simulink model "eightenPulseRectifier"  (R2024a)
settings: Solver=VariableStepAuto  StartTime=0.0  StopTime=.1  MaxStep=.00001  RelTol=1e-3
undefined symbols (not defined in the file): D1, lagging, pulse
libraries: spsVoltageMeasurementLib x34, spsControlledVoltageSourceLib x9, spsUniversalBridgeLib x9, spsSeriesRLCBranchLib x6, spsZigzagPhaseShiftingTransformerLib x6, spsGroundLib x5, spsThreePhaseTransformerTwoWindingsLib x3, spsPulseGeneratorThyristor6PulseLib x2, spsPLLLib x1, spsPLL3phLib x1, spsRMSLib x1, spsThreePhaseVIMeasurementLib x1
settings Model: Creator=User  LastModifiedBy=User

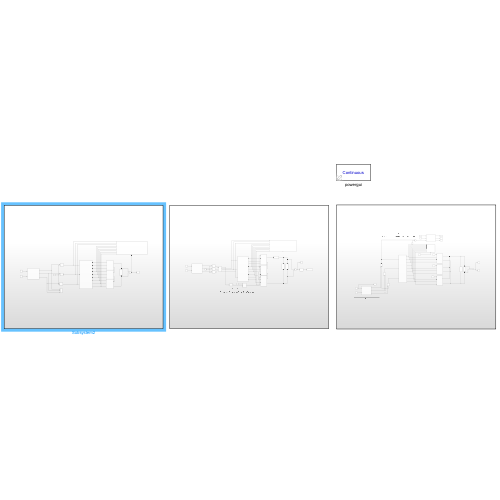
[thumbnail: Simulink's stored preview of the top-level diagram]
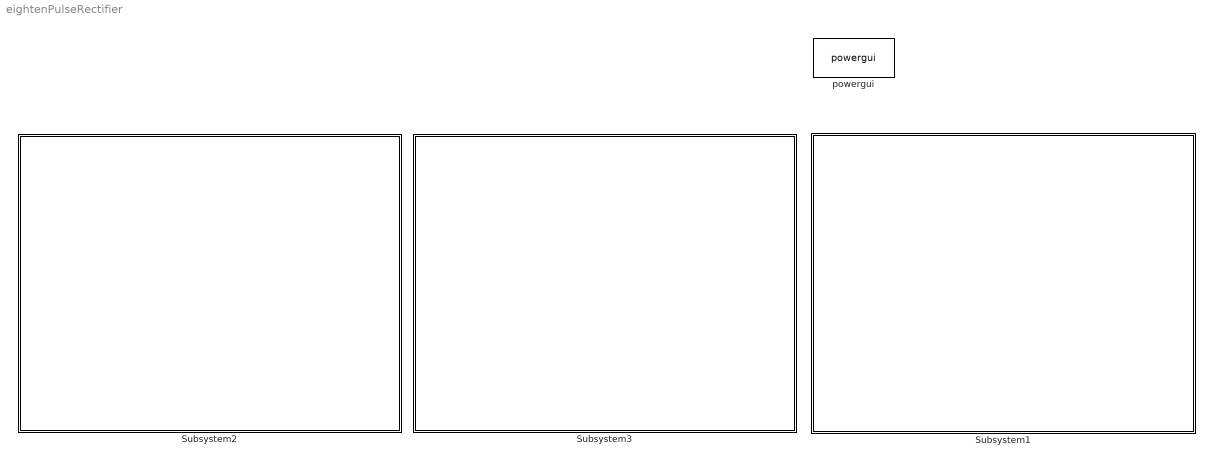
== system eightenPulseRectifier ==
  Subsystem1 : Subsystem
  Subsystem2 : Subsystem
  Subsystem3 : Subsystem
  powergui : sps_lib/powergui  Priority=1  SimulationMode=Continuous  SampleTime=50e-6  frequency=60  Iterations=50  frequencyindice=0  Pbase=100e6  ErrMax=1e-4  UnitsV=kV  UnitsW=MW  buscounter=0  FunctionMessages=off  echomessages=off  EnableUseOfTLC=off  CurrentSourceSwitches=off  DisableSnubberDevices=off  DisableRonSwitches=off  DisableVfSwitches=off  DisplayEquations=off  AutomaticDiscreteSolvers=off  SolverType=Tustin/Backward Euler (TBE)  Interpol=off  ExternalGateDelay=off  methode=off  Ts=100  x0status=blocks  SPID=on  SwTol=0  HookPort=off  NonlinearTolerance=1e-4  nMaxIteration=100  ContinueOnMaxIteration=off  RestoreLinks=warning  ResistiveCurrentMeasurement=off  Frange=[0:2:500]  Ylog=off  Xlog=on  ShowGrid=off  save=off  variable=ZData  structure=0  ZoomFFT=off  StartTime=0.0  cycles=1  DisplayStyle=1  fundamental=60  FreqAxis=off  MaxFrequency=1000  frequencyindicesteady=1  RmsSteady=1  display=off

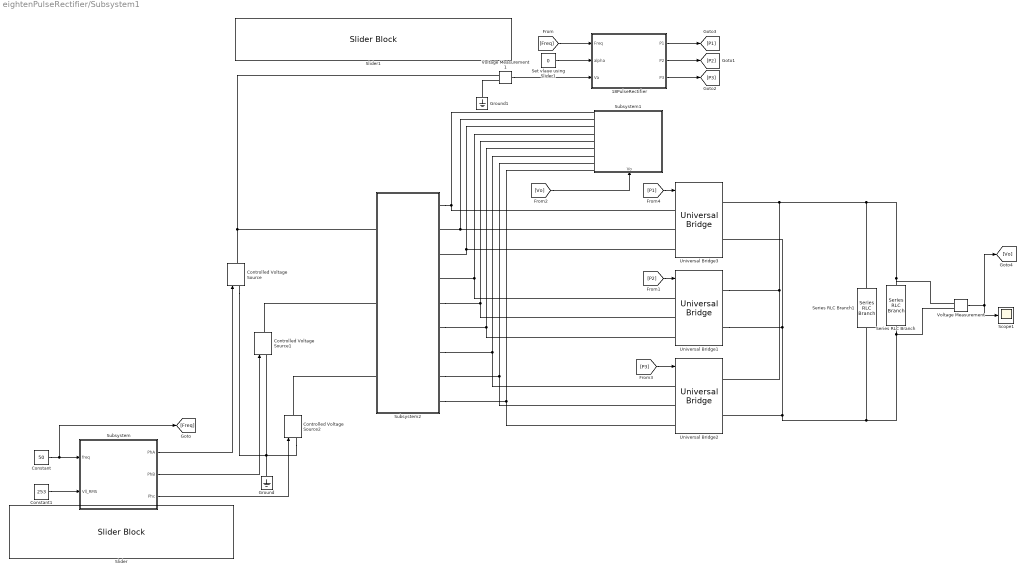
== system eightenPulseRectifier/Subsystem1 ==
  18PulseRectifier : Subsystem
  Constant : Constant  Value=50
  Constant1 : Constant  Value=253
  Controlled Voltage Source : spsControlledVoltageSourceLib/Controlled Voltage Source  Initialize=on  Source_Type=AC  Amplitude=0  Phase=0  Frequency=0  Measurements=None
  Controlled Voltage Source1 : spsControlledVoltageSourceLib/Controlled Voltage Source  Initialize=on  Source_Type=AC  Amplitude=0  Phase=0  Frequency=0  Measurements=None
  Controlled Voltage Source2 : spsControlledVoltageSourceLib/Controlled Voltage Source  Initialize=on  Source_Type=AC  Amplitude=0  Phase=0  Frequency=0  Measurements=None
  Ground : spsGroundLib/Ground  LConnTagsString=a
  Ground1 : spsGroundLib/Ground  LConnTagsString=a
  Scope1 : Scope
  Series RLC Branch : spsSeriesRLCBranchLib/Series RLC Branch  LConnTagsString=__new0  RConnTagsString=__new0  BranchType=R  Resistance=1  Inductance=1e-3  SetiL0=off  InitialCurrent=0  Capacitance=1e-6  Setx0=off  InitialVoltage=0  Measurements=None
  Series RLC Branch1 : spsSeriesRLCBranchLib/Series RLC Branch  LConnTagsString=__new0  RConnTagsString=__new0  BranchType=C  Resistance=1  Inductance=1e-3  SetiL0=off  InitialCurrent=0  Capacitance=1e-6  Setx0=off  InitialVoltage=0  Measurements=None
  Set vlaue using Slider1 : Constant  Value=0
  Slider : SliderBlock  ScaleMin=187  ScaleMax=253
  Slider1 : SliderBlock  ScaleMax=150  TickInterval=5
  Subsystem : Subsystem
  Subsystem1 : Subsystem
      settings: PortSchema="{\"entries\":[{\"content\":{\"sides\":[{\"content\":{\"connectorIds\":[\"LConn1\",\"LConn2\",\"LConn3\",\"LConn4\",\"LConn5\",\"LConn6\",\"LConn7\",\"LConn8\",\"LConn9\"]},\"type\":\"ConnectorPlacement.EquallySpacedRectSide\",\"uuid\":\"c528b960-0f89-4916-bc59-feafc106a6fa\"},{\"content\":{\"side\":\"RIGHT\"},\"type\":\"ConnectorPlacement.EquallySpacedRectSide\",\"uuid\":\"71a864a5-f7f4-48a7-95f9-d8a7d95b84d2\"},{\"content\":{\"side\":\"TOP\"},\"type\":\"ConnectorPlacement.EquallySpacedRectSide\",\"uuid\":\"57c5c08c-8233-4b40-a9fb-e09e67286da5\"},{\"content\":{\"connectorIds\":[\"In1\"],\"side\":\"BOTTOM\"},\"type\":\"ConnectorPlacement.EquallySpacedRectSide\",\"uuid\":\"030adcd8-0531-402c-81c9-62e294f4d5af\"}]},\"type\":\"ConnectorPlacement.EquallySpacedConnector\",\"uuid\":\"216ad3eb-0ca6-4d39-b862-04814928268f\"}],\"packageUris\":[\"http://schema.mathworks.com/mf0/Connector/R2020b\"],\"version\":\"1.0\"}"
  Subsystem2 : Subsystem
  Universal Bridge1 : spsUniversalBridgeLib/Universal Bridge  Arms=3  SnubberResistance=1e5  SnubberCapacitance=inf  Device=Thyristors  Ron=1e-3  Lon=0  ForwardVoltages="[  0  0  ]"  ForwardVoltage=0  GTOparameters=[ 10e-6 , 20e-6 ]  IGBTparameters=[ 1e-6 , 2e-6 ]  Measurements=None  Measurements_2=None  converterType=Rectifier
  Universal Bridge2 : spsUniversalBridgeLib/Universal Bridge  Arms=3  SnubberResistance=1e5  SnubberCapacitance=inf  Device=Thyristors  Ron=1e-3  Lon=0  ForwardVoltages="[  0  0  ]"  ForwardVoltage=0  GTOparameters=[ 10e-6 , 20e-6 ]  IGBTparameters=[ 1e-6 , 2e-6 ]  Measurements=None  Measurements_2=None  converterType=Rectifier
  Universal Bridge3 : spsUniversalBridgeLib/Universal Bridge  Arms=3  SnubberResistance=1e5  SnubberCapacitance=inf  Device=Thyristors  Ron=1e-3  Lon=0  ForwardVoltages="[  0  0  ]"  ForwardVoltage=0  GTOparameters=[ 10e-6 , 20e-6 ]  IGBTparameters=[ 1e-6 , 2e-6 ]  Measurements=None  Measurements_2=None  converterType=Rectifier
  Voltage Measurement : spsVoltageMeasurementLib/Voltage Measurement  PhasorSimulation=off  OutputType=Complex  PSBequivalent=0
  Voltage Measurement1 : spsVoltageMeasurementLib/Voltage Measurement  PhasorSimulation=off  OutputType=Complex  PSBequivalent=0
  wires:
  Constant/1 -> [Freq], Subsystem/1(freq)
  Constant1/1 -> Subsystem/2(Vll_RMS)
  Subsystem/3(Phc) -> Controlled Voltage Source2/1
  Subsystem/2(PhB) -> Controlled Voltage Source1/1
  Subsystem/1(PhA) -> Controlled Voltage Source/1
  [P3] -> Universal Bridge2/1
  [Freq] -> 18PulseRectifier/1(Freq)
  18PulseRectifier/1(P1) -> [P1]
  18PulseRectifier/2(P2) -> [P2]
  18PulseRectifier/3(P3) -> [P3]
  Set vlaue using Slider1/1 -> 18PulseRectifier/2(alpha)
  Voltage Measurement/1 -> Scope1/1, [Vo]
  [Vo] -> Subsystem1/1(Vo)
  [P1] -> Universal Bridge3/1
  [P2] -> Universal Bridge1/1
  Voltage Measurement1/1 -> 18PulseRectifier/3(Va)
  connections:
  Subsystem1/LConn9 -- Universal Bridge2/LConn3 -- Subsystem2/RConn9
  Subsystem1/LConn6 -- Universal Bridge1/LConn3 -- Subsystem2/RConn6
  Controlled Voltage Source/RConn1 -- Voltage Measurement1/LConn1 -- Subsystem2/LConn1
  Subsystem1/LConn5 -- Universal Bridge1/LConn2 -- Subsystem2/RConn5
  Subsystem1/LConn7 -- Universal Bridge2/LConn1 -- Subsystem2/RConn7
  Subsystem1/LConn3 -- Subsystem2/RConn3 -- Universal Bridge3/LConn3
  Ground/LConn1 -- Controlled Voltage Source1/LConn1 -- Controlled Voltage Source/LConn1 -- Controlled Voltage Source2/LConn1
  Subsystem1/LConn2 -- Subsystem2/RConn2 -- Universal Bridge3/LConn2
  Voltage Measurement/LConn1 -- Series RLC Branch1/LConn1 -- Universal Bridge2/RConn1 -- Universal Bridge1/RConn1 -- Universal Bridge3/RConn1 -- Series RLC Branch/LConn1
  Series RLC Branch/RConn1 -- Universal Bridge1/RConn2 -- Universal Bridge3/RConn2 -- Universal Bridge2/RConn2 -- Series RLC Branch1/RConn1 -- Voltage Measurement/LConn2
  Subsystem1/LConn8 -- Universal Bridge2/LConn2 -- Subsystem2/RConn8
  Subsystem1/LConn4 -- Universal Bridge1/LConn1 -- Subsystem2/RConn4
  Controlled Voltage Source2/RConn1 -- Subsystem2/LConn3
  Controlled Voltage Source1/RConn1 -- Subsystem2/LConn2
  Subsystem1/LConn1 -- Universal Bridge3/LConn1 -- Subsystem2/RConn1
  Ground1/LConn1 -- Voltage Measurement1/LConn2

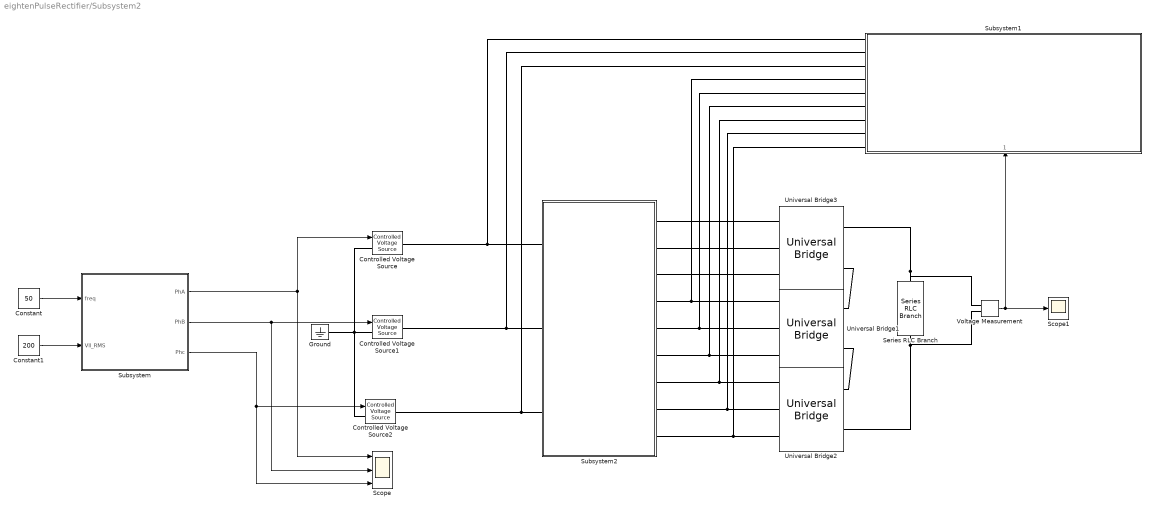
== system eightenPulseRectifier/Subsystem2 ==
  Constant : Constant  Value=50
  Constant1 : Constant  Value=200
  Controlled Voltage Source : spsControlledVoltageSourceLib/Controlled Voltage Source  Initialize=on  Source_Type=AC  Amplitude=0  Phase=0  Frequency=0  Measurements=None
  Controlled Voltage Source1 : spsControlledVoltageSourceLib/Controlled Voltage Source  Initialize=on  Source_Type=AC  Amplitude=0  Phase=0  Frequency=0  Measurements=None
  Controlled Voltage Source2 : spsControlledVoltageSourceLib/Controlled Voltage Source  Initialize=on  Source_Type=AC  Amplitude=0  Phase=0  Frequency=0  Measurements=None
  Ground : spsGroundLib/Ground  LConnTagsString=a
  Scope : Scope  NumInputPorts=3
  Scope1 : Scope
  Series RLC Branch : spsSeriesRLCBranchLib/Series RLC Branch  LConnTagsString=__new0  RConnTagsString=__new0  BranchType=R  Resistance=20  Inductance=1e-3  SetiL0=off  InitialCurrent=0  Capacitance=1e-6  Setx0=off  InitialVoltage=0  Measurements=None
  Subsystem : Subsystem
  Subsystem1 : Subsystem
      settings: PortSchema="{\"entries\":[{\"content\":{\"sides\":[{\"content\":{\"connectorIds\":[\"LConn1\",\"LConn2\",\"LConn3\",\"LConn4\",\"LConn5\",\"LConn6\",\"LConn7\",\"LConn8\",\"LConn9\"]},\"type\":\"ConnectorPlacement.EquallySpacedRectSide\",\"uuid\":\"c528b960-0f89-4916-bc59-feafc106a6fa\"},{\"content\":{\"side\":\"RIGHT\"},\"type\":\"ConnectorPlacement.EquallySpacedRectSide\",\"uuid\":\"71a864a5-f7f4-48a7-95f9-d8a7d95b84d2\"},{\"content\":{\"side\":\"TOP\"},\"type\":\"ConnectorPlacement.EquallySpacedRectSide\",\"uuid\":\"57c5c08c-8233-4b40-a9fb-e09e67286da5\"},{\"content\":{\"connectorIds\":[\"In1\"],\"side\":\"BOTTOM\"},\"type\":\"ConnectorPlacement.EquallySpacedRectSide\",\"uuid\":\"f6f9f7ac-8837-43ce-91db-f6801ff1a468\"}]},\"type\":\"ConnectorPlacement.EquallySpacedConnector\",\"uuid\":\"216ad3eb-0ca6-4d39-b862-04814928268f\"}],\"packageUris\":[\"http://schema.mathworks.com/mf0/Connector/R2020b\"],\"version\":\"1.0\"}"
  Subsystem2 : Subsystem
  Universal Bridge1 : spsUniversalBridgeLib/Universal Bridge  Arms=3  SnubberResistance=1e5  SnubberCapacitance=inf  Device=Diodes  Ron=1e-3  Lon=0  ForwardVoltages="[  0  0  ]"  ForwardVoltage=0  GTOparameters=[ 10e-6 , 20e-6 ]  IGBTparameters=[ 1e-6 , 2e-6 ]  Measurements=None  Measurements_2=None  converterType=Rectifier
  Universal Bridge2 : spsUniversalBridgeLib/Universal Bridge  Arms=3  SnubberResistance=1e5  SnubberCapacitance=inf  Device=Diodes  Ron=1e-3  Lon=0  ForwardVoltages="[  0  0  ]"  ForwardVoltage=0  GTOparameters=[ 10e-6 , 20e-6 ]  IGBTparameters=[ 1e-6 , 2e-6 ]  Measurements=None  Measurements_2=None  converterType=Rectifier
  Universal Bridge3 : spsUniversalBridgeLib/Universal Bridge  Arms=3  SnubberResistance=1e5  SnubberCapacitance=inf  Device=Diodes  Ron=1e-3  Lon=0  ForwardVoltages="[  0  0  ]"  ForwardVoltage=0  GTOparameters=[ 10e-6 , 20e-6 ]  IGBTparameters=[ 1e-6 , 2e-6 ]  Measurements=None  Measurements_2=None  converterType=Rectifier
  Voltage Measurement : spsVoltageMeasurementLib/Voltage Measurement  PhasorSimulation=off  OutputType=Complex  PSBequivalent=0
  wires:
  Subsystem/1(PhA) -> Controlled Voltage Source/1, Scope/1
  Subsystem/2(PhB) -> Scope/2, Controlled Voltage Source1/1
  Subsystem/3(Phc) -> Scope/3, Controlled Voltage Source2/1
  Constant1/1 -> Subsystem/2(Vll_RMS)
  Constant/1 -> Subsystem/1(freq)
  Voltage Measurement/1 -> Scope1/1, Subsystem1/1(" ")
  connections:
  Subsystem2/RConn3 -- Universal Bridge3/LConn3
  Subsystem2/RConn2 -- Universal Bridge3/LConn2
  Subsystem2/RConn1 -- Universal Bridge3/LConn1
  Subsystem2/RConn7 -- Subsystem1/LConn7 -- Universal Bridge2/LConn1
  Subsystem1/LConn2 -- Subsystem2/LConn2 -- Controlled Voltage Source1/RConn1
  Subsystem2/RConn9 -- Subsystem1/LConn9 -- Universal Bridge2/LConn3
  Subsystem2/RConn6 -- Universal Bridge1/LConn3 -- Subsystem1/LConn6
  Subsystem2/LConn1 -- Controlled Voltage Source/RConn1 -- Subsystem1/LConn1
  Subsystem2/LConn3 -- Controlled Voltage Source2/RConn1 -- Subsystem1/LConn3
  Subsystem2/RConn8 -- Subsystem1/LConn8 -- Universal Bridge2/LConn2
  Subsystem2/RConn4 -- Universal Bridge1/LConn1 -- Subsystem1/LConn4
  Controlled Voltage Source1/LConn1 -- Controlled Voltage Source2/LConn1 -- Ground/LConn1 -- Controlled Voltage Source/LConn1
  Subsystem2/RConn5 -- Universal Bridge1/LConn2 -- Subsystem1/LConn5
  Voltage Measurement/LConn1 -- Universal Bridge3/RConn1 -- Series RLC Branch/LConn1
  Universal Bridge3/RConn2 -- Universal Bridge1/RConn1
  Universal Bridge1/RConn2 -- Universal Bridge2/RConn1
  Voltage Measurement/LConn2 -- Universal Bridge2/RConn2 -- Series RLC Branch/RConn1

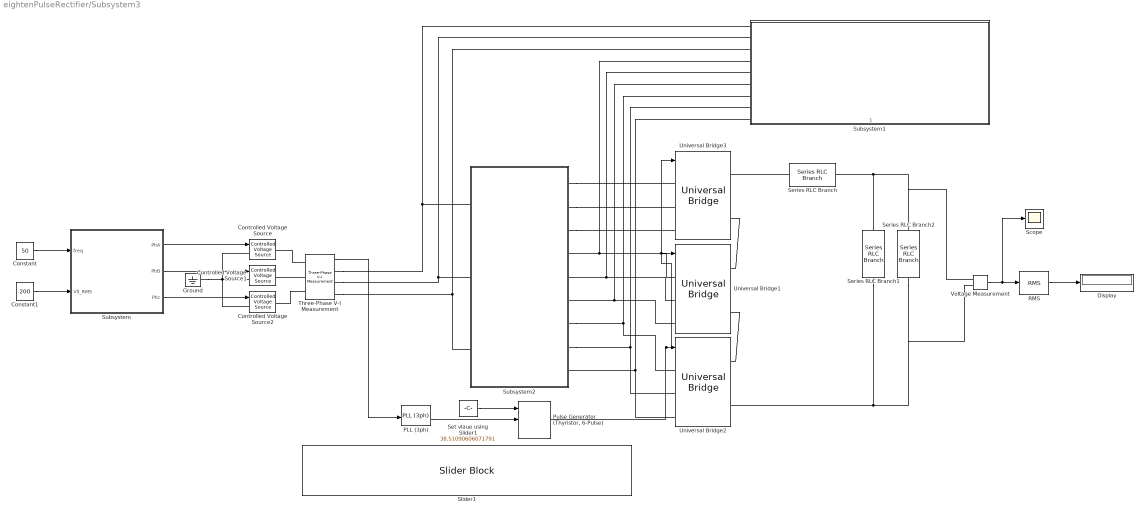
== system eightenPulseRectifier/Subsystem3 ==
  Constant : Constant  Value=50
  Constant1 : Constant  Value=200
  Controlled Voltage Source : spsControlledVoltageSourceLib/Controlled Voltage Source  Initialize=on  Source_Type=AC  Amplitude=0  Phase=0  Frequency=0  Measurements=None
  Controlled Voltage Source1 : spsControlledVoltageSourceLib/Controlled Voltage Source  Initialize=on  Source_Type=AC  Amplitude=0  Phase=0  Frequency=0  Measurements=None
  Controlled Voltage Source2 : spsControlledVoltageSourceLib/Controlled Voltage Source  Initialize=on  Source_Type=AC  Amplitude=0  Phase=0  Frequency=0  Measurements=None
  Display : Display
  Ground : spsGroundLib/Ground  LConnTagsString=a
  PLL (3ph) : spsPLL3phLib/PLL (3ph)  Fmin=45  Par_Init=[0, 60]  ParK=[180, 3200, 1]  TcD=1e-4  MaxRateChangeFreq=12  FilterCutOffFreq=25  Ts=0  AGC=on
  "Pulse Generator (Thyristor, 6-Pulse)" : spsPulseGeneratorThyristor6PulseLib/Pulse Generator (Thyristor, 6-Pulse)  GenType=6-pulse  Delta=D1 (lagging)  pwidth=120  Double_Pulse=off  Ts=0
      settings: LibrarySourceBlock=|
      | sps_lib/Power Electronics/Power Electronics Control/Pulse Generator
      | (Thyristor, 6-Pulse)
  RMS : spsRMSLib/RMS  TrueRMS=on  Freq=50  RMSInit=120  Ts=0
  Scope : Scope
  Series RLC Branch : spsSeriesRLCBranchLib/Series RLC Branch  LConnTagsString=__new0  RConnTagsString=__new0  BranchType=L  Resistance=1  Inductance=200e-3  SetiL0=off  InitialCurrent=0  Capacitance=1e-6  Setx0=off  InitialVoltage=0  Measurements=None
  Series RLC Branch1 : spsSeriesRLCBranchLib/Series RLC Branch  LConnTagsString=__new0  RConnTagsString=__new0  BranchType=C  Resistance=1  Inductance=200e-3  SetiL0=off  InitialCurrent=0  Capacitance=10e-6  Setx0=off  InitialVoltage=0  Measurements=None
  Series RLC Branch2 : spsSeriesRLCBranchLib/Series RLC Branch  LConnTagsString=__new0  RConnTagsString=__new0  BranchType=R  Resistance=1400  Inductance=200e-3  SetiL0=off  InitialCurrent=0  Capacitance=10e-6  Setx0=off  InitialVoltage=0  Measurements=None
  Set vlaue using Slider1 : Constant  Value=38.51090606071791
  Slider1 : SliderBlock  ScaleMax=150  TickInterval=5
  Subsystem : Subsystem
  Subsystem1 : Subsystem
      settings: PortSchema="{\"entries\":[{\"content\":{\"sides\":[{\"content\":{\"connectorIds\":[\"LConn1\",\"LConn2\",\"LConn3\",\"LConn4\",\"LConn5\",\"LConn6\",\"LConn7\",\"LConn8\",\"LConn9\"]},\"type\":\"ConnectorPlacement.EquallySpacedRectSide\",\"uuid\":\"c528b960-0f89-4916-bc59-feafc106a6fa\"},{\"content\":{\"side\":\"RIGHT\"},\"type\":\"ConnectorPlacement.EquallySpacedRectSide\",\"uuid\":\"71a864a5-f7f4-48a7-95f9-d8a7d95b84d2\"},{\"content\":{\"side\":\"TOP\"},\"type\":\"ConnectorPlacement.EquallySpacedRectSide\",\"uuid\":\"57c5c08c-8233-4b40-a9fb-e09e67286da5\"},{\"content\":{\"connectorIds\":[\"In1\"],\"side\":\"BOTTOM\"},\"type\":\"ConnectorPlacement.EquallySpacedRectSide\",\"uuid\":\"f6f9f7ac-8837-43ce-91db-f6801ff1a468\"}]},\"type\":\"ConnectorPlacement.EquallySpacedConnector\",\"uuid\":\"216ad3eb-0ca6-4d39-b862-04814928268f\"}],\"packageUris\":[\"http://schema.mathworks.com/mf0/Connector/R2020b\"],\"version\":\"1.0\"}"
  Subsystem2 : Subsystem
  Three-Phase V-I Measurement : spsThreePhaseVIMeasurementLib/Three-Phase V-I Measurement  VoltageMeasurement=phase-to-ground  SetLabelV=off  LabelV=Vabc  Vpu=off  VpuLL=off  CurrentMeasurement=no  SetLabelI=off  LabelI=Iabc  Ipu=off  Pbase=100e6  Vbase=500e3  OutputType=Complex  PhasorSimulation=off  PSBequivalent=0
  Universal Bridge1 : spsUniversalBridgeLib/Universal Bridge  Arms=3  SnubberResistance=1e5  SnubberCapacitance=inf  Device=Thyristors  Ron=1e-3  Lon=0  ForwardVoltages="[  0  0  ]"  ForwardVoltage=0  GTOparameters=[ 10e-6 , 20e-6 ]  IGBTparameters=[ 1e-6 , 2e-6 ]  Measurements=None  Measurements_2=None  converterType=Rectifier
  Universal Bridge2 : spsUniversalBridgeLib/Universal Bridge  Arms=3  SnubberResistance=1e5  SnubberCapacitance=inf  Device=Thyristors  Ron=1e-3  Lon=0  ForwardVoltages="[  0  0  ]"  ForwardVoltage=0  GTOparameters=[ 10e-6 , 20e-6 ]  IGBTparameters=[ 1e-6 , 2e-6 ]  Measurements=None  Measurements_2=None  converterType=Rectifier
  Universal Bridge3 : spsUniversalBridgeLib/Universal Bridge  Arms=3  SnubberResistance=1e5  SnubberCapacitance=inf  Device=Thyristors  Ron=1e-3  Lon=0  ForwardVoltages="[  0  0  ]"  ForwardVoltage=0  GTOparameters=[ 10e-6 , 20e-6 ]  IGBTparameters=[ 1e-6 , 2e-6 ]  Measurements=None  Measurements_2=None  converterType=Rectifier
  Voltage Measurement : spsVoltageMeasurementLib/Voltage Measurement  PhasorSimulation=off  OutputType=Complex  PSBequivalent=0
  wires:
  Constant/1 -> Subsystem/1(freq)
  Constant1/1 -> Subsystem/2(Vll_RMS)
  Subsystem/3(Phc) -> Controlled Voltage Source2/1
  Subsystem/2(PhB) -> Controlled Voltage Source1/1
  Subsystem/1(PhA) -> Controlled Voltage Source/1
  Three-Phase V-I Measurement/1 -> PLL (3ph)/1
  PLL (3ph)/2 -> "Pulse Generator (Thyristor, 6-Pulse)"/2
  Set vlaue using Slider1/1 -> "Pulse Generator (Thyristor, 6-Pulse)"/1
  "Pulse Generator (Thyristor, 6-Pulse)"/1 -> Universal Bridge3/1, Universal Bridge1/1, Universal Bridge2/1
  Voltage Measurement/1 -> Scope/1, RMS/1
  RMS/1 -> Display/1
  connections:
  Subsystem1/LConn5 -- Universal Bridge1/LConn2 -- Subsystem2/RConn5
  Ground/LConn1 -- Controlled Voltage Source/LConn1 -- Controlled Voltage Source1/LConn1 -- Controlled Voltage Source2/LConn1
  Subsystem1/LConn4 -- Universal Bridge1/LConn1 -- Subsystem2/RConn4
  Subsystem1/LConn8 -- Universal Bridge2/LConn2 -- Subsystem2/RConn8
  Subsystem1/LConn3 -- Subsystem2/LConn3 -- Three-Phase V-I Measurement/RConn3
  Subsystem1/LConn1 -- Three-Phase V-I Measurement/RConn1 -- Subsystem2/LConn1
  Subsystem1/LConn6 -- Universal Bridge1/LConn3 -- Subsystem2/RConn6
  Subsystem1/LConn9 -- Universal Bridge2/LConn3 -- Subsystem2/RConn9
  Subsystem2/LConn2 -- Subsystem1/LConn2 -- Three-Phase V-I Measurement/RConn2
  Subsystem1/LConn7 -- Universal Bridge2/LConn1 -- Subsystem2/RConn7
  Subsystem2/RConn1 -- Universal Bridge3/LConn1
  Subsystem2/RConn2 -- Universal Bridge3/LConn2
  Subsystem2/RConn3 -- Universal Bridge3/LConn3
  Three-Phase V-I Measurement/LConn1 -- Controlled Voltage Source/RConn1
  Three-Phase V-I Measurement/LConn2 -- Controlled Voltage Source1/RConn1
  Three-Phase V-I Measurement/LConn3 -- Controlled Voltage Source2/RConn1
  Universal Bridge3/RConn2 -- Universal Bridge1/RConn1
  Universal Bridge1/RConn2 -- Universal Bridge2/RConn1
  Series RLC Branch/LConn1 -- Universal Bridge3/RConn1
  Series RLC Branch1/LConn1 -- Voltage Measurement/LConn1 -- Series RLC Branch2/LConn1 -- Series RLC Branch/RConn1
  Series RLC Branch1/RConn1 -- Series RLC Branch2/RConn1 -- Voltage Measurement/LConn2 -- Universal Bridge2/RConn2

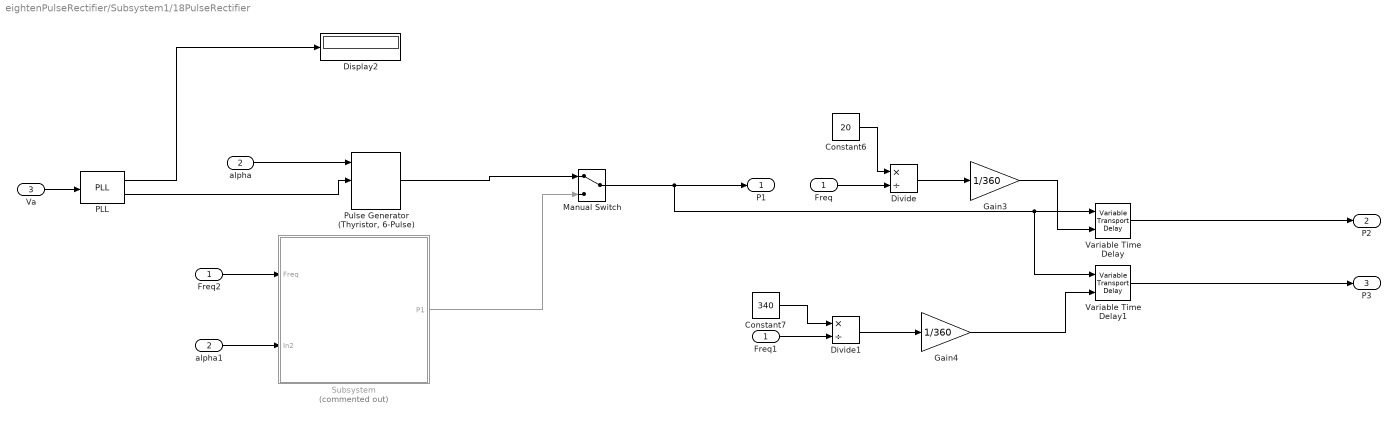
== system eightenPulseRectifier/Subsystem1/18PulseRectifier ==
  Freq : Inport
  alpha : Inport  Port=2
  Va : Inport  Port=3
  Constant6 : Constant  Value=20
  Constant7 : Constant  Value=340
  Display2 : Display
  Divide : Product  Inputs=*/
  Divide1 : Product  Inputs=*/
  Freq1 : InportShadow
  Freq2 : InportShadow
  Gain3 : Gain  Gain=1/360
  Gain4 : Gain  Gain=1/360
  Manual Switch : ManualSwitch
  PLL : spsPLLLib/PLL  Fmin=45  Par_Init=[0, 60]  ParK=[180, 3200, 1]  TcD=1e-4  MaxRateChangeFreq=12  FilterCutOffFreq=25  Ts=0  AGC=on
      settings: LibrarySourceBlock=sps_lib/Control/PLL
  "Pulse Generator (Thyristor, 6-Pulse)" : spsPulseGeneratorThyristor6PulseLib/Pulse Generator (Thyristor, 6-Pulse)  GenType=6-pulse  Delta=D1 (lagging)  pwidth=60  Double_Pulse=off  Ts=0
      settings: LibrarySourceBlock=|
      | sps_lib/Power Electronics/Power Electronics Control/Pulse Generator
      | (Thyristor, 6-Pulse)
  Subsystem : Subsystem  Commented=on
  Variable Time Delay : VariableTransportDelay  MaximumDelay=10
  Variable Time Delay1 : VariableTransportDelay  MaximumDelay=10
  alpha1 : InportShadow  Port=2
  P1 : Outport
  P2 : Outport  Port=2
  P3 : Outport  Port=3
  wires:
  Divide1/1 -> Gain4/1
  Gain4/1 -> Variable Time Delay1/2
  Divide/1 -> Gain3/1
  Gain3/1 -> Variable Time Delay/2
  Variable Time Delay1/1 -> P3/1
  Constant7/1 -> Divide1/1
  Variable Time Delay/1 -> P2/1
  Constant6/1 -> Divide/1
  Freq/1 -> Divide/2
  Freq1/1 -> Divide1/2
  alpha/1 -> "Pulse Generator (Thyristor, 6-Pulse)"/1
  PLL/2 -> "Pulse Generator (Thyristor, 6-Pulse)"/2
  PLL/1 -> Display2/1
  Va/1 -> PLL/1
  Freq2/1 -> Subsystem/1(Freq)
  alpha1/1 -> Subsystem/2(In2)
  Subsystem/1(P1) -> Manual Switch/2
  "Pulse Generator (Thyristor, 6-Pulse)"/1 -> Manual Switch/1
  Manual Switch/1 -> P1/1, Variable Time Delay1/1, Variable Time Delay/1

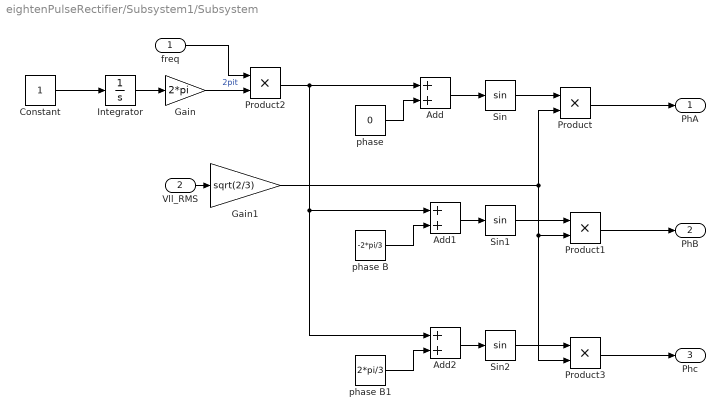
== system eightenPulseRectifier/Subsystem1/Subsystem ==
  freq : Inport
  Vll_RMS : Inport  Port=2
  Add : Sum
  Add1 : Sum
  Add2 : Sum
  Constant : Constant
  Gain : Gain  Gain=2*pi
  Gain1 : Gain  Gain=sqrt(2/3)
  Integrator : Integrator
  Product{,1..3} (4 alike) : Product
  Sin : Trigonometry
  Sin1 : Trigonometry
  Sin2 : Trigonometry
  phase : Constant  Value=0
  phase B : Constant  Value=-2*pi/3
  phase B1 : Constant  Value=2*pi/3
  PhA : Outport
  PhB : Outport  Port=2
  Phc : Outport  Port=3
  wires:
  Sin/1 -> Product/1
  Product3/1 -> Phc/1
  freq/1 -> Product2/1
  Product/1 -> PhA/1
  phase B1/1 -> Add2/2
  Add2/1 -> Sin2/1
  Add1/1 -> Sin1/1
  Add/1 -> Sin/1
  phase B/1 -> Add1/2
  phase/1 -> Add/2
  Vll_RMS/1 -> Gain1/1
  Constant/1 -> Integrator/1
  Integrator/1 -> Gain/1
  Product2/1 -> Add/1, Add1/1, Add2/1
  Product1/1 -> PhB/1
  Sin2/1 -> Product3/1
  Sin1/1 -> Product1/1
  Gain/1 -> Product2/2  "2pit"
  Gain1/1 -> Product1/2, Product3/2, Product/2

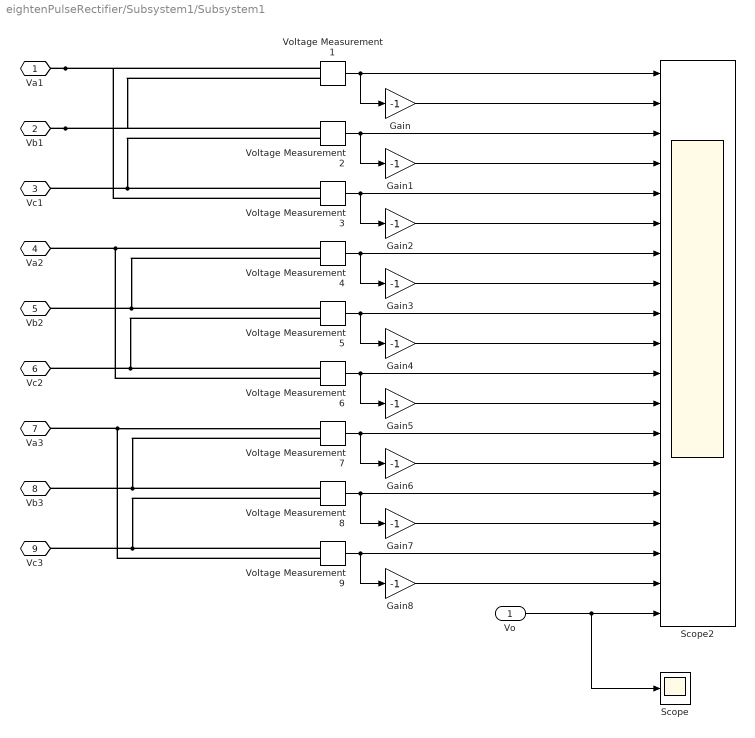
== system eightenPulseRectifier/Subsystem1/Subsystem1 ==
  Vo : Inport
  Gain{,1..8} (9 alike) : Gain  Gain=-1
  Scope : Scope
  Scope2 : Scope  NumInputPorts=19
  Voltage Measurement{1..9} (9 alike) : spsVoltageMeasurementLib/Voltage Measurement  PhasorSimulation=off  OutputType=Complex  PSBequivalent=0
  Va1 : PMIOPort  Side=Left
  Vb1 : PMIOPort  Port=2  Side=Left
  Vc1 : PMIOPort  Port=3  Side=Left
  Va2 : PMIOPort  Port=4  Side=Left
  Vb2 : PMIOPort  Port=5  Side=Left
  Vc2 : PMIOPort  Port=6  Side=Left
  Va3 : PMIOPort  Port=7  Side=Left
  Vb3 : PMIOPort  Port=8  Side=Left
  Vc3 : PMIOPort  Port=9  Side=Left
  wires:
  Voltage Measurement2/1 -> Gain1/1, Scope2/3
  Voltage Measurement4/1 -> Gain3/1, Scope2/7
  Voltage Measurement5/1 -> Gain4/1, Scope2/9
  Voltage Measurement3/1 -> Gain2/1, Scope2/5
  Gain1/1 -> Scope2/4
  Gain8/1 -> Scope2/18
  Gain7/1 -> Scope2/16
  Voltage Measurement9/1 -> Gain8/1, Scope2/17
  Gain5/1 -> Scope2/12
  Voltage Measurement7/1 -> Gain6/1, Scope2/13
  Voltage Measurement6/1 -> Gain5/1, Scope2/11
  Voltage Measurement1/1 -> Gain/1, Scope2/1
  Voltage Measurement8/1 -> Gain7/1, Scope2/15
  Gain4/1 -> Scope2/10
  Gain2/1 -> Scope2/6
  Gain/1 -> Scope2/2
  Gain6/1 -> Scope2/14
  Gain3/1 -> Scope2/8
  Vo/1 -> Scope/1, Scope2/19
  connections:
  Voltage Measurement6/LConn1 -- Voltage Measurement5/LConn2 -- Vc2/RConn1
  Voltage Measurement9/LConn1 -- Voltage Measurement8/LConn2 -- Vc3/RConn1
  Voltage Measurement5/LConn1 -- Voltage Measurement4/LConn2 -- Vb2/RConn1
  Va1/RConn1 -- Voltage Measurement1/LConn1 -- Voltage Measurement3/LConn2
  Voltage Measurement4/LConn1 -- Voltage Measurement6/LConn2 -- Va2/RConn1
  Voltage Measurement9/LConn2 -- Va3/RConn1 -- Voltage Measurement7/LConn1
  Voltage Measurement3/LConn1 -- Voltage Measurement2/LConn2 -- Vc1/RConn1
  Vb1/RConn1 -- Voltage Measurement2/LConn1 -- Voltage Measurement1/LConn2
  Voltage Measurement8/LConn1 -- Voltage Measurement7/LConn2 -- Vb3/RConn1

== system eightenPulseRectifier/Subsystem1/Subsystem2 ==
  Three-Phase Transformer (Two Windings) : spsThreePhaseTransformerTwoWindingsLib/Three-Phase Transformer (Two Windings)  Winding1Connection=Yg  Winding2Connection=Yg  CoreType=Three single-phase transformers  SetSaturation=off  Hysteresis=off  DataFile='hysteresis'  SetInitialFlux=off  Measurements=None  UNITS=SI  NominalPower=[ 250e6 , 50 ]  Winding1=[253/sqrt(3) 0 0]  Winding2=[253/sqrt(3) 0 0]  Rm=1.0804e+06  Lm=2866  L0=0.5  Saturation=[0 0;0.66653 1910.3;277.72 2419.7]  InitialFluxes=[ 0.8 , -0.8 , 0.7 ]  BreakLoop=off  DiscreteSolver=Trapezoidal iterative  DataType=on  TransfoNumber=1
  Zigzag Phase-Shifting Transformer : spsZigzagPhaseShiftingTransformerLib/Zigzag Phase-Shifting Transformer  SecondaryConnection=Yg  SetSaturation=off  SetInitialFlux=off  Measurements=None  UNITS=SI  NominalPower=[ 100e6 50]  PrimaryVoltage=200/sqrt(3)  SecondaryVoltage="[ 200/sqrt(3)  +20]"  Winding1=[0.002488 0.00026399]  Winding2=[0.00017863 1.8954e-05]  Winding3=[0.018 0.0019099]  RmLm=[622.01 1.6499]  Rm=622.01  Saturation=[0 0;17.569 28.988;7320.5 36.718]  InitialFluxes=[0 0 0]  BreakLoop=off  DiscreteSolver=Trapezoidal iterative  DataType=on
      settings: LibrarySourceBlock=|
      | sps_lib/Power Grid Elements/Zigzag
      | Phase-Shifting Transformer
  Zigzag Phase-Shifting Transformer2 : spsZigzagPhaseShiftingTransformerLib/Zigzag Phase-Shifting Transformer  SecondaryConnection=Yg  SetSaturation=off  SetInitialFlux=off  Measurements=None  UNITS=SI  NominalPower=[ 100e6 50]  PrimaryVoltage=200/sqrt(3)  SecondaryVoltage="[ 200/sqrt(3)  -20]"  Winding1=[0.002488 0.00026399]  Winding2=[0.00017863 1.8954e-05]  Winding3=[0.018 0.0019099]  RmLm=[622.01 1.6499]  Rm=622.01  Saturation=[0 0;17.569 28.988;7320.5 36.718]  InitialFluxes=[0 0 0]  BreakLoop=off  DiscreteSolver=Trapezoidal iterative  DataType=on
      settings: LibrarySourceBlock=|
      | sps_lib/Power Grid Elements/Zigzag
      | Phase-Shifting Transformer
  A : PMIOPort  Side=Left
  B : PMIOPort  Port=2  Side=Left
  C : PMIOPort  Port=3  Side=Left
  R1 : PMIOPort  Port=4  Side=Right
  S1 : PMIOPort  Port=5  Side=Right
  T1 : PMIOPort  Port=6  Side=Right
  R2 : PMIOPort  Port=7  Side=Right
  S2 : PMIOPort  Port=8  Side=Right
  T2 : PMIOPort  Port=9  Side=Right
  R3 : PMIOPort  Port=10  Side=Right
  S3 : PMIOPort  Port=11  Side=Right
  T3 : PMIOPort  Port=12  Side=Right
  connections:
  Zigzag Phase-Shifting Transformer2/LConn1 -- R3/RConn1
  Zigzag Phase-Shifting Transformer2/LConn5 -- Zigzag Phase-Shifting Transformer2/LConn6 -- Zigzag Phase-Shifting Transformer2/LConn4
  R2/RConn1 -- Zigzag Phase-Shifting Transformer/LConn1
  Zigzag Phase-Shifting Transformer/LConn5 -- Zigzag Phase-Shifting Transformer/LConn4 -- Zigzag Phase-Shifting Transformer/LConn6
  Zigzag Phase-Shifting Transformer/RConn1 -- A/RConn1 -- Three-Phase Transformer (Two Windings)/LConn1 -- Zigzag Phase-Shifting Transformer2/RConn1
  T3/RConn1 -- Zigzag Phase-Shifting Transformer2/LConn3
  Three-Phase Transformer (Two Windings)/RConn3 -- T1/RConn1
  Zigzag Phase-Shifting Transformer2/LConn2 -- S3/RConn1
  T2/RConn1 -- Zigzag Phase-Shifting Transformer/LConn3
  Zigzag Phase-Shifting Transformer/RConn2 -- B/RConn1 -- Three-Phase Transformer (Two Windings)/LConn2 -- Zigzag Phase-Shifting Transformer2/RConn2
  S2/RConn1 -- Zigzag Phase-Shifting Transformer/LConn2
  Three-Phase Transformer (Two Windings)/RConn2 -- S1/RConn1
  Three-Phase Transformer (Two Windings)/RConn1 -- R1/RConn1
  C/RConn1 -- Three-Phase Transformer (Two Windings)/LConn3 -- Zigzag Phase-Shifting Transformer2/RConn3 -- Zigzag Phase-Shifting Transformer/RConn3

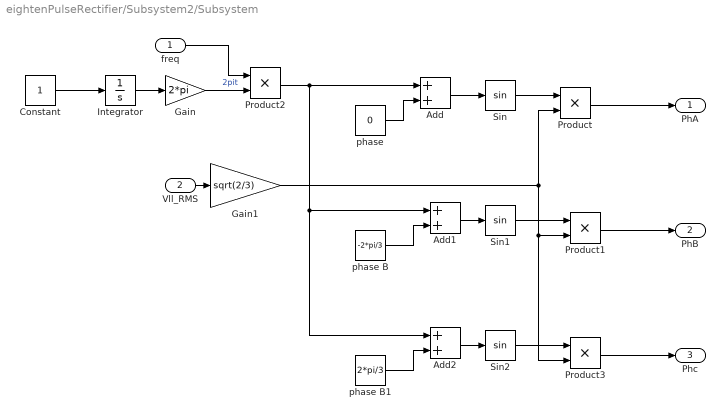
== system eightenPulseRectifier/Subsystem2/Subsystem ==
  freq : Inport
  Vll_RMS : Inport  Port=2
  Add : Sum
  Add1 : Sum
  Add2 : Sum
  Constant : Constant
  Gain : Gain  Gain=2*pi
  Gain1 : Gain  Gain=sqrt(2/3)
  Integrator : Integrator
  Product{,1..3} (4 alike) : Product
  Sin : Trigonometry
  Sin1 : Trigonometry
  Sin2 : Trigonometry
  phase : Constant  Value=0
  phase B : Constant  Value=-2*pi/3
  phase B1 : Constant  Value=2*pi/3
  PhA : Outport
  PhB : Outport  Port=2
  Phc : Outport  Port=3
  wires:
  Gain1/1 -> Product/2, Product3/2, Product1/2
  Gain/1 -> Product2/2  "2pit"
  Sin1/1 -> Product1/1
  Sin2/1 -> Product3/1
  Product1/1 -> PhB/1
  Product2/1 -> Add2/1, Add1/1, Add/1
  Integrator/1 -> Gain/1
  Constant/1 -> Integrator/1
  Vll_RMS/1 -> Gain1/1
  phase/1 -> Add/2
  phase B/1 -> Add1/2
  Add/1 -> Sin/1
  Add1/1 -> Sin1/1
  Add2/1 -> Sin2/1
  phase B1/1 -> Add2/2
  Product/1 -> PhA/1
  freq/1 -> Product2/1
  Product3/1 -> Phc/1
  Sin/1 -> Product/1

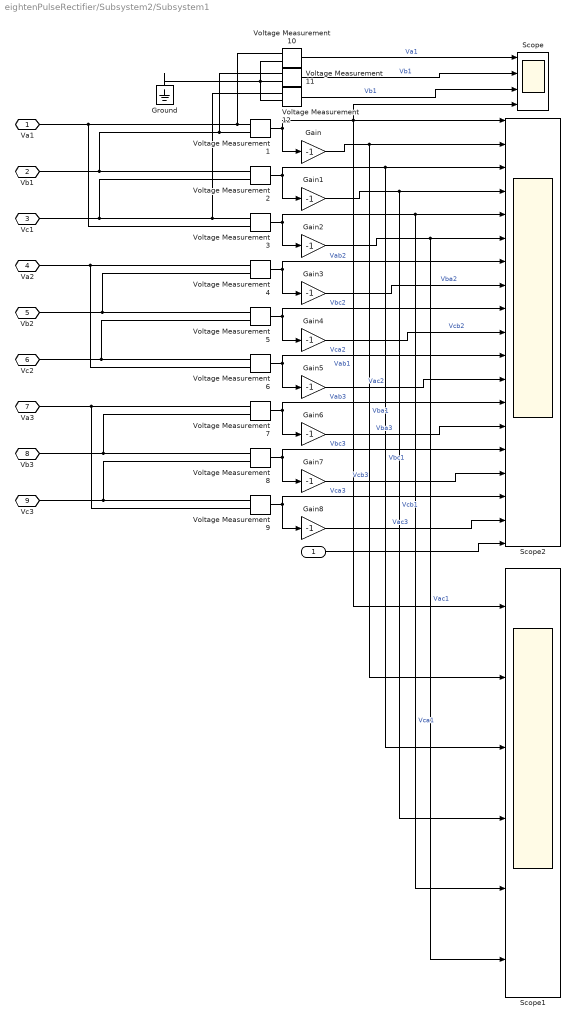
== system eightenPulseRectifier/Subsystem2/Subsystem1 ==
  " " : Inport
  Gain{,1..8} (9 alike) : Gain  Gain=-1
  Ground : spsGroundLib/Ground  LConnTagsString=a
  Scope : Scope  NumInputPorts=4
  Scope1 : Scope  NumInputPorts=6
  Scope2 : Scope  NumInputPorts=19
  Voltage Measurement{1..12} (12 alike) : spsVoltageMeasurementLib/Voltage Measurement  PhasorSimulation=off  OutputType=Complex  PSBequivalent=0
  Va1 : PMIOPort  Side=Left
  Vb1 : PMIOPort  Port=2  Side=Left
  Vc1 : PMIOPort  Port=3  Side=Left
  Va2 : PMIOPort  Port=4  Side=Left
  Vb2 : PMIOPort  Port=5  Side=Left
  Vc2 : PMIOPort  Port=6  Side=Left
  Va3 : PMIOPort  Port=7  Side=Left
  Vb3 : PMIOPort  Port=8  Side=Left
  Vc3 : PMIOPort  Port=9  Side=Left
  wires:
  " "/1 -> Scope2/19
  Voltage Measurement2/1 -> Gain1/1, Scope1/3, Scope2/3  "Vbc1"
  Voltage Measurement4/1 -> Gain3/1, Scope2/7  "Vab2"
  Voltage Measurement5/1 -> Gain4/1, Scope2/9  "Vbc2"
  Voltage Measurement3/1 -> Gain2/1, Scope1/5, Scope2/5  "Vca1"
  Gain1/1 -> Scope1/4, Scope2/4  "Vcb1"
  Gain8/1 -> Scope2/18  "Vac3"
  Gain7/1 -> Scope2/16  "Vcb3"
  Voltage Measurement9/1 -> Gain8/1, Scope2/17  "Vca3"
  Gain5/1 -> Scope2/12  "Vac2"
  Voltage Measurement7/1 -> Gain6/1, Scope2/13  "Vab3"
  Voltage Measurement6/1 -> Gain5/1, Scope2/11  "Vca2"
  Voltage Measurement1/1 -> Gain/1, Scope/4, Scope1/1, Scope2/1  "Vab1"
  Voltage Measurement8/1 -> Gain7/1, Scope2/15  "Vbc3"
  Gain4/1 -> Scope2/10  "Vcb2"
  Gain2/1 -> Scope1/6, Scope2/6  "Vac1"
  Gain/1 -> Scope1/2, Scope2/2  "Vba1"
  Gain6/1 -> Scope2/14  "Vba3"
  Gain3/1 -> Scope2/8  "Vba2"
  Voltage Measurement10/1 -> Scope/1  "Va1"
  Voltage Measurement11/1 -> Scope/2  "Vb1"
  Voltage Measurement12/1 -> Scope/3  "Vb1"
  connections:
  Voltage Measurement6/LConn1 -- Voltage Measurement5/LConn2 -- Vc2/RConn1
  Voltage Measurement8/LConn2 -- Voltage Measurement9/LConn1 -- Vc3/RConn1
  Voltage Measurement5/LConn1 -- Voltage Measurement4/LConn2 -- Vb2/RConn1
  Voltage Measurement1/LConn1 -- Voltage Measurement3/LConn2 -- Va1/RConn1 -- Voltage Measurement10/LConn1
  Voltage Measurement6/LConn2 -- Voltage Measurement4/LConn1 -- Va2/RConn1
  Voltage Measurement9/LConn2 -- Voltage Measurement7/LConn1 -- Va3/RConn1
  Voltage Measurement2/LConn2 -- Voltage Measurement12/LConn1 -- Voltage Measurement3/LConn1 -- Vc1/RConn1
  Voltage Measurement2/LConn1 -- Voltage Measurement1/LConn2 -- Voltage Measurement11/LConn1 -- Vb1/RConn1
  Voltage Measurement7/LConn2 -- Voltage Measurement8/LConn1 -- Vb3/RConn1
  Ground/LConn1 -- Voltage Measurement10/LConn2 -- Voltage Measurement12/LConn2 -- Voltage Measurement11/LConn2

== system eightenPulseRectifier/Subsystem2/Subsystem2 ==
  Three-Phase Transformer (Two Windings) : spsThreePhaseTransformerTwoWindingsLib/Three-Phase Transformer (Two Windings)  Winding1Connection=Yg  Winding2Connection=Yg  CoreType=Three single-phase transformers  SetSaturation=off  Hysteresis=off  DataFile='hysteresis'  SetInitialFlux=off  Measurements=None  UNITS=SI  NominalPower=[ 250e6 , 50 ]  Winding1=[253/sqrt(3) 0 0]  Winding2=[253/sqrt(3) 0 0]  Rm=1.0804e+06  Lm=2866  L0=0.5  Saturation=[0 0;0.66653 1910.3;277.72 2419.7]  InitialFluxes=[ 0.8 , -0.8 , 0.7 ]  BreakLoop=off  DiscreteSolver=Trapezoidal iterative  DataType=on  TransfoNumber=1
  Zigzag Phase-Shifting Transformer : spsZigzagPhaseShiftingTransformerLib/Zigzag Phase-Shifting Transformer  SecondaryConnection=Yg  SetSaturation=off  SetInitialFlux=off  Measurements=None  UNITS=SI  NominalPower=[ 100e6 50]  PrimaryVoltage=200/sqrt(3)  SecondaryVoltage="[ 200/sqrt(3)  +20]"  Winding1=[0.002488 0.00026399]  Winding2=[0.00017863 1.8954e-05]  Winding3=[0.018 0.0019099]  RmLm=[622.01 1.6499]  Rm=622.01  Saturation=[0 0;17.569 28.988;7320.5 36.718]  InitialFluxes=[0 0 0]  BreakLoop=off  DiscreteSolver=Trapezoidal iterative  DataType=on
      settings: LibrarySourceBlock=|
      | sps_lib/Power Grid Elements/Zigzag
      | Phase-Shifting Transformer
  Zigzag Phase-Shifting Transformer2 : spsZigzagPhaseShiftingTransformerLib/Zigzag Phase-Shifting Transformer  SecondaryConnection=Yg  SetSaturation=off  SetInitialFlux=off  Measurements=None  UNITS=SI  NominalPower=[ 100e6 50]  PrimaryVoltage=200/sqrt(3)  SecondaryVoltage="[ 200/sqrt(3)  -20]"  Winding1=[0.002488 0.00026399]  Winding2=[0.00017863 1.8954e-05]  Winding3=[0.018 0.0019099]  RmLm=[622.01 1.6499]  Rm=622.01  Saturation=[0 0;17.569 28.988;7320.5 36.718]  InitialFluxes=[0 0 0]  BreakLoop=off  DiscreteSolver=Trapezoidal iterative  DataType=on
      settings: LibrarySourceBlock=|
      | sps_lib/Power Grid Elements/Zigzag
      | Phase-Shifting Transformer
  A : PMIOPort  Side=Left
  B : PMIOPort  Port=2  Side=Left
  C : PMIOPort  Port=3  Side=Left
  R1 : PMIOPort  Port=4  Side=Right
  S1 : PMIOPort  Port=5  Side=Right
  T1 : PMIOPort  Port=6  Side=Right
  R2 : PMIOPort  Port=7  Side=Right
  S2 : PMIOPort  Port=8  Side=Right
  T2 : PMIOPort  Port=9  Side=Right
  R3 : PMIOPort  Port=10  Side=Right
  S3 : PMIOPort  Port=11  Side=Right
  T3 : PMIOPort  Port=12  Side=Right
  connections:
  Zigzag Phase-Shifting Transformer/RConn3 -- Zigzag Phase-Shifting Transformer2/RConn3 -- Three-Phase Transformer (Two Windings)/LConn3 -- C/RConn1
  Three-Phase Transformer (Two Windings)/RConn1 -- R1/RConn1
  Three-Phase Transformer (Two Windings)/RConn2 -- S1/RConn1
  S2/RConn1 -- Zigzag Phase-Shifting Transformer/LConn2
  Zigzag Phase-Shifting Transformer2/RConn2 -- Three-Phase Transformer (Two Windings)/LConn2 -- B/RConn1 -- Zigzag Phase-Shifting Transformer/RConn2
  T2/RConn1 -- Zigzag Phase-Shifting Transformer/LConn3
  Zigzag Phase-Shifting Transformer2/LConn2 -- S3/RConn1
  Three-Phase Transformer (Two Windings)/RConn3 -- T1/RConn1
  T3/RConn1 -- Zigzag Phase-Shifting Transformer2/LConn3
  Zigzag Phase-Shifting Transformer2/RConn1 -- Three-Phase Transformer (Two Windings)/LConn1 -- A/RConn1 -- Zigzag Phase-Shifting Transformer/RConn1
  Zigzag Phase-Shifting Transformer/LConn6 -- Zigzag Phase-Shifting Transformer/LConn4 -- Zigzag Phase-Shifting Transformer/LConn5
  R2/RConn1 -- Zigzag Phase-Shifting Transformer/LConn1
  Zigzag Phase-Shifting Transformer2/LConn4 -- Zigzag Phase-Shifting Transformer2/LConn6 -- Zigzag Phase-Shifting Transformer2/LConn5
  Zigzag Phase-Shifting Transformer2/LConn1 -- R3/RConn1

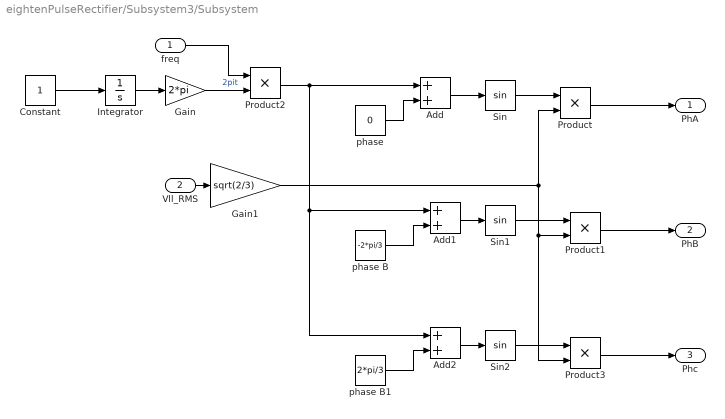
== system eightenPulseRectifier/Subsystem3/Subsystem ==
  freq : Inport
  Vll_RMS : Inport  Port=2
  Add : Sum
  Add1 : Sum
  Add2 : Sum
  Constant : Constant
  Gain : Gain  Gain=2*pi
  Gain1 : Gain  Gain=sqrt(2/3)
  Integrator : Integrator
  Product{,1..3} (4 alike) : Product
  Sin : Trigonometry
  Sin1 : Trigonometry
  Sin2 : Trigonometry
  phase : Constant  Value=0
  phase B : Constant  Value=-2*pi/3
  phase B1 : Constant  Value=2*pi/3
  PhA : Outport
  PhB : Outport  Port=2
  Phc : Outport  Port=3
  wires:
  Sin/1 -> Product/1
  Product3/1 -> Phc/1
  freq/1 -> Product2/1
  Product/1 -> PhA/1
  phase B1/1 -> Add2/2
  Add2/1 -> Sin2/1
  Add1/1 -> Sin1/1
  Add/1 -> Sin/1
  phase B/1 -> Add1/2
  phase/1 -> Add/2
  Vll_RMS/1 -> Gain1/1
  Constant/1 -> Integrator/1
  Integrator/1 -> Gain/1
  Product2/1 -> Add/1, Add1/1, Add2/1
  Product1/1 -> PhB/1
  Sin2/1 -> Product3/1
  Sin1/1 -> Product1/1
  Gain/1 -> Product2/2  "2pit"
  Gain1/1 -> Product1/2, Product3/2, Product/2

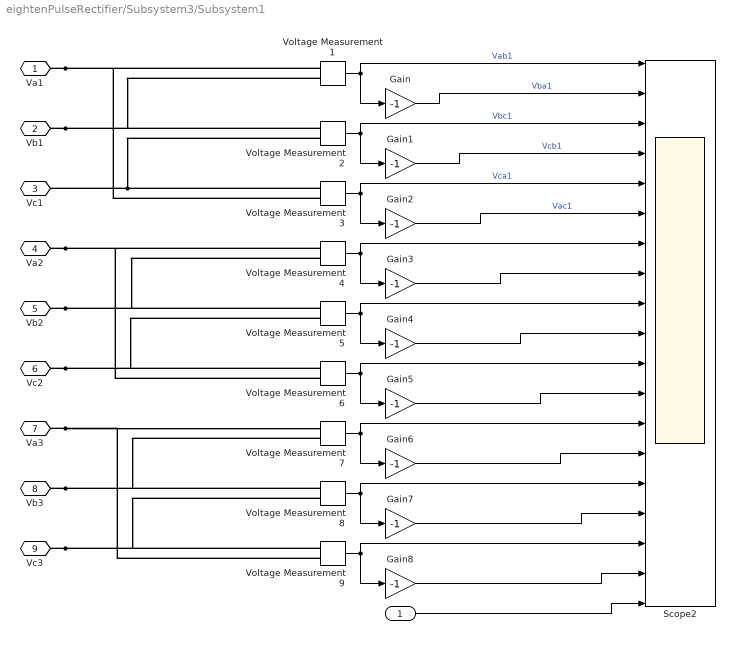
== system eightenPulseRectifier/Subsystem3/Subsystem1 ==
  " " : Inport
  Gain{,1..8} (9 alike) : Gain  Gain=-1
  Scope2 : Scope  NumInputPorts=19
  Voltage Measurement{1..9} (9 alike) : spsVoltageMeasurementLib/Voltage Measurement  PhasorSimulation=off  OutputType=Complex  PSBequivalent=0
  Va1 : PMIOPort  Side=Left
  Vb1 : PMIOPort  Port=2  Side=Left
  Vc1 : PMIOPort  Port=3  Side=Left
  Va2 : PMIOPort  Port=4  Side=Left
  Vb2 : PMIOPort  Port=5  Side=Left
  Vc2 : PMIOPort  Port=6  Side=Left
  Va3 : PMIOPort  Port=7  Side=Left
  Vb3 : PMIOPort  Port=8  Side=Left
  Vc3 : PMIOPort  Port=9  Side=Left
  wires:
  Gain3/1 -> Scope2/8
  Gain6/1 -> Scope2/14
  Gain/1 -> Scope2/2  "Vba1"
  Gain2/1 -> Scope2/6  "Vac1"
  Gain4/1 -> Scope2/10
  Voltage Measurement8/1 -> Scope2/15, Gain7/1
  Voltage Measurement1/1 -> Scope2/1, Gain/1  "Vab1"
  Voltage Measurement6/1 -> Scope2/11, Gain5/1
  Voltage Measurement7/1 -> Scope2/13, Gain6/1
  Gain5/1 -> Scope2/12
  Voltage Measurement9/1 -> Scope2/17, Gain8/1
  Gain7/1 -> Scope2/16
  Gain8/1 -> Scope2/18
  Gain1/1 -> Scope2/4  "Vcb1"
  Voltage Measurement3/1 -> Scope2/5, Gain2/1  "Vca1"
  Voltage Measurement5/1 -> Scope2/9, Gain4/1
  Voltage Measurement4/1 -> Scope2/7, Gain3/1
  Voltage Measurement2/1 -> Scope2/3, Gain1/1  "Vbc1"
  " "/1 -> Scope2/19
  connections:
  Vb3/RConn1 -- Voltage Measurement8/LConn1 -- Voltage Measurement7/LConn2
  Vb1/RConn1 -- Voltage Measurement1/LConn2 -- Voltage Measurement2/LConn1
  Voltage Measurement3/LConn1 -- Vc1/RConn1 -- Voltage Measurement2/LConn2
  Va3/RConn1 -- Voltage Measurement7/LConn1 -- Voltage Measurement9/LConn2
  Va2/RConn1 -- Voltage Measurement4/LConn1 -- Voltage Measurement6/LConn2
  Va1/RConn1 -- Voltage Measurement3/LConn2 -- Voltage Measurement1/LConn1
  Vb2/RConn1 -- Voltage Measurement4/LConn2 -- Voltage Measurement5/LConn1
  Vc3/RConn1 -- Voltage Measurement9/LConn1 -- Voltage Measurement8/LConn2
  Vc2/RConn1 -- Voltage Measurement5/LConn2 -- Voltage Measurement6/LConn1

== system eightenPulseRectifier/Subsystem3/Subsystem2 ==
  Three-Phase Transformer (Two Windings) : spsThreePhaseTransformerTwoWindingsLib/Three-Phase Transformer (Two Windings)  Winding1Connection=Yg  Winding2Connection=Yg  CoreType=Three single-phase transformers  SetSaturation=off  Hysteresis=off  DataFile='hysteresis'  SetInitialFlux=off  Measurements=None  UNITS=SI  NominalPower=[ 250e6 , 50 ]  Winding1=[253/sqrt(3) 0 0]  Winding2=[253/sqrt(3) 0 0]  Rm=1.0804e+06  Lm=2866  L0=0.5  Saturation=[0 0;0.66653 1910.3;277.72 2419.7]  InitialFluxes=[ 0.8 , -0.8 , 0.7 ]  BreakLoop=off  DiscreteSolver=Trapezoidal iterative  DataType=on  TransfoNumber=1
  Zigzag Phase-Shifting Transformer : spsZigzagPhaseShiftingTransformerLib/Zigzag Phase-Shifting Transformer  SecondaryConnection=Yg  SetSaturation=off  SetInitialFlux=off  Measurements=None  UNITS=SI  NominalPower=[ 100e6 50]  PrimaryVoltage=200/sqrt(3)  SecondaryVoltage="[ 200/sqrt(3)  +20]"  Winding1=[0.002488 0.00026399]  Winding2=[0.00017863 1.8954e-05]  Winding3=[0.018 0.0019099]  RmLm=[622.01 1.6499]  Rm=622.01  Saturation=[0 0;17.569 28.988;7320.5 36.718]  InitialFluxes=[0 0 0]  BreakLoop=off  DiscreteSolver=Trapezoidal iterative  DataType=on
      settings: LibrarySourceBlock=|
      | sps_lib/Power Grid Elements/Zigzag
      | Phase-Shifting Transformer
  Zigzag Phase-Shifting Transformer2 : spsZigzagPhaseShiftingTransformerLib/Zigzag Phase-Shifting Transformer  SecondaryConnection=Yg  SetSaturation=off  SetInitialFlux=off  Measurements=None  UNITS=SI  NominalPower=[ 100e6 50]  PrimaryVoltage=200/sqrt(3)  SecondaryVoltage="[ 200/sqrt(3)  -20]"  Winding1=[0.002488 0.00026399]  Winding2=[0.00017863 1.8954e-05]  Winding3=[0.018 0.0019099]  RmLm=[622.01 1.6499]  Rm=622.01  Saturation=[0 0;17.569 28.988;7320.5 36.718]  InitialFluxes=[0 0 0]  BreakLoop=off  DiscreteSolver=Trapezoidal iterative  DataType=on
      settings: LibrarySourceBlock=|
      | sps_lib/Power Grid Elements/Zigzag
      | Phase-Shifting Transformer
  A : PMIOPort  Side=Left
  B : PMIOPort  Port=2  Side=Left
  C : PMIOPort  Port=3  Side=Left
  R1 : PMIOPort  Port=4  Side=Right
  S1 : PMIOPort  Port=5  Side=Right
  T1 : PMIOPort  Port=6  Side=Right
  R2 : PMIOPort  Port=7  Side=Right
  S2 : PMIOPort  Port=8  Side=Right
  T2 : PMIOPort  Port=9  Side=Right
  R3 : PMIOPort  Port=10  Side=Right
  S3 : PMIOPort  Port=11  Side=Right
  T3 : PMIOPort  Port=12  Side=Right
  connections:
  Zigzag Phase-Shifting Transformer2/LConn1 -- R3/RConn1
  Zigzag Phase-Shifting Transformer2/LConn6 -- Zigzag Phase-Shifting Transformer2/LConn5 -- Zigzag Phase-Shifting Transformer2/LConn4
  R2/RConn1 -- Zigzag Phase-Shifting Transformer/LConn1
  Zigzag Phase-Shifting Transformer/LConn5 -- Zigzag Phase-Shifting Transformer/LConn6 -- Zigzag Phase-Shifting Transformer/LConn4
  Three-Phase Transformer (Two Windings)/LConn1 -- Zigzag Phase-Shifting Transformer2/RConn1 -- Zigzag Phase-Shifting Transformer/RConn1 -- A/RConn1
  T3/RConn1 -- Zigzag Phase-Shifting Transformer2/LConn3
  Three-Phase Transformer (Two Windings)/RConn3 -- T1/RConn1
  Zigzag Phase-Shifting Transformer2/LConn2 -- S3/RConn1
  T2/RConn1 -- Zigzag Phase-Shifting Transformer/LConn3
  Three-Phase Transformer (Two Windings)/LConn2 -- Zigzag Phase-Shifting Transformer2/RConn2 -- Zigzag Phase-Shifting Transformer/RConn2 -- B/RConn1
  S2/RConn1 -- Zigzag Phase-Shifting Transformer/LConn2
  Three-Phase Transformer (Two Windings)/RConn2 -- S1/RConn1
  Three-Phase Transformer (Two Windings)/RConn1 -- R1/RConn1
  Three-Phase Transformer (Two Windings)/LConn3 -- Zigzag Phase-Shifting Transformer2/RConn3 -- Zigzag Phase-Shifting Transformer/RConn3 -- C/RConn1

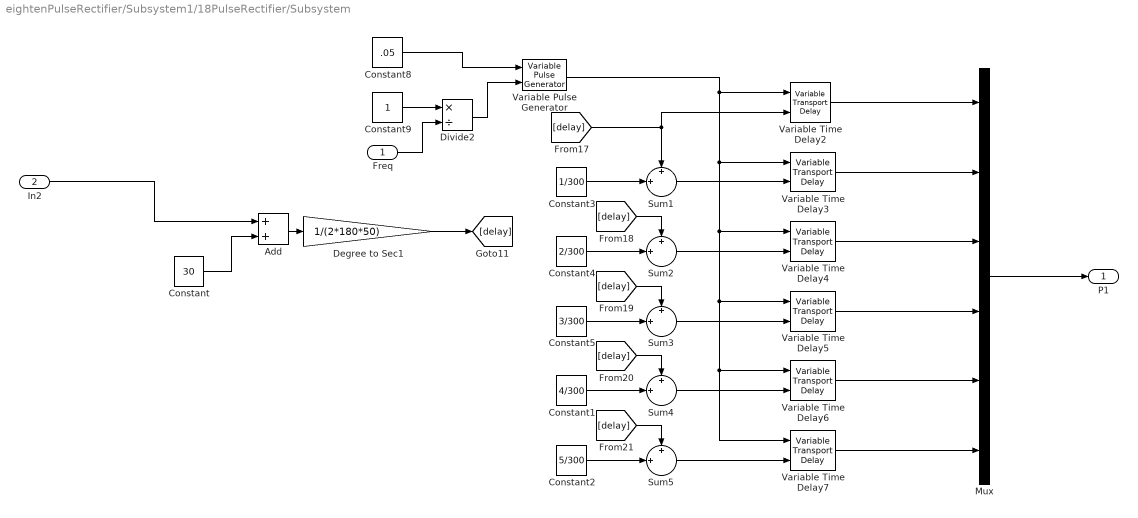
== system eightenPulseRectifier/Subsystem1/18PulseRectifier/Subsystem ==
  Freq : Inport
  In2 : Inport  Port=2
  Add : Sum
  Constant : Constant  Value=30
  Constant1 : Constant  Value=4/300
  Constant2 : Constant  Value=5/300
  Constant3 : Constant  Value=1/300
  Constant4 : Constant  Value=2/300
  Constant5 : Constant  Value=3/300
  Constant8 : Constant  Value=.05
  Constant9 : Constant
  Degree to Sec1 : Gain  Gain=1/(2*180*50)
  Divide2 : Product  Inputs=*/
  Mux : Mux  Inputs=6
  Sum{1..5} (5 alike) : Sum  Inputs=+|+||
  Variable Time Delay{2..7} (6 alike) : VariableTransportDelay  MaximumDelay=10
  Variable Pulse Generator : VariablePulseGenerator  SampleTime=0.1
  P1 : Outport
  wires:
  Variable Time Delay7/1 -> Mux/6
  Freq/1 -> Divide2/2
  Constant/1 -> Add/2
  Sum4/1 -> Variable Time Delay6/2
  Variable Time Delay4/1 -> Mux/3
  Constant4/1 -> Sum2/2
  [delay] -> Sum4/1
  Sum5/1 -> Variable Time Delay7/2
  Variable Time Delay3/1 -> Mux/2
  Constant8/1 -> Variable Pulse Generator/1
  Constant1/1 -> Sum4/2
  Divide2/1 -> Variable Pulse Generator/2
  Degree to Sec1/1 -> [delay]
  Constant9/1 -> Divide2/1
  Variable Time Delay5/1 -> Mux/4
  Variable Pulse Generator/1 -> Variable Time Delay4/1, Variable Time Delay5/1, Variable Time Delay6/1, Variable Time Delay7/1, Variable Time Delay3/1, Variable Time Delay2/1
  [delay] -> Variable Time Delay2/2, Sum1/1
  [delay] -> Sum3/1
  Variable Time Delay2/1 -> Mux/1
  Sum1/1 -> Variable Time Delay3/2
  [delay] -> Sum2/1
  Sum2/1 -> Variable Time Delay4/2
  Sum3/1 -> Variable Time Delay5/2
  Constant5/1 -> Sum3/2
  In2/1 -> Add/1
  [delay] -> Sum5/1
  Constant2/1 -> Sum5/2
  Variable Time Delay6/1 -> Mux/5
  Constant3/1 -> Sum1/2
  Add/1 -> Degree to Sec1/1
  Mux/1 -> P1/1
